simulink model "Discrete_Time_rising_ic_verif"  (Simulink 8.4)
settings: Solver=ode45  StartTime=0.0  StopTime=10.0  RelTol=1e-3
undefined symbols (not defined in the file): DiscIntNeverNeededParam, sigbuilder_block
settings Model: Creator=Romain  LastModifiedBy=hbourbou
settings DataIOCC: SignalLoggingSaveFormat=Dataset
settings OptimizationCC: ExpressionDepthLimit=128
settings DebuggingCC: SolverPrmCheckMsg=none  FcnCallInpInsideContextMsg=EnableAllAsError  FrameProcessingCompatibilityMsg=error  StateNameClashWarn=none
settings GRTTargetCC: CombineOutputUpdateFcns=on  GRTInterface=off

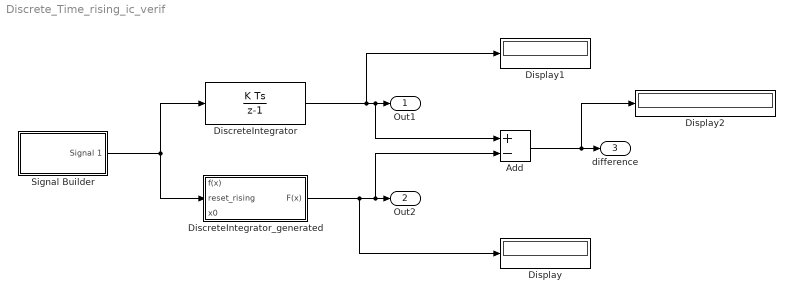
== system Discrete_Time_rising_ic_verif ==
  Add : Sum  Inputs=+-
  DiscreteIntegrator : DiscreteIntegrator  ExternalReset=rising  InitialConditionSource=external  InitialConditionSetting=State (most efficient)  SampleTime=-1  ICPrevOutput=DiscIntNeverNeededParam  ICPrevScaledInput=DiscIntNeverNeededParam
  DiscreteIntegrator_generated : Subsystem  TreatAsAtomicUnit=on
  Display : Display
  Display1 : Display
  Display2 : Display
  Signal Builder : Subsystem  Tag=STV Subsys  LoadFcn=sigbuilder_block('load');  StartFcn=sigbuilder_block('start');  StopFcn=sigbuilder_block('stop');  ClipboardFcn=sigbuilder_block('clipboard');  mask(Sigbuilder block){}
      mask help: Simulink:masks:SigbuilderBlock_MD
      mask init:
      | if ~strcmp(get_param(bdroot(gcbh),'SimulationStatus'),'stopped') tuvar = sigbuilder_block('maskInit'); end
      settings: CopyFcn=sigbuilder_block('copy');  DeleteFcn=sigbuilder_block('delete');  ModelCloseFcn=sigbuilder_block('modelClose');  PreSaveFcn=sigbuilder_block('preSave');  PauseFcn=sigbuilder_block('pause');  ContinueFcn=sigbuilder_block('continue');  NameChangeFcn=sigbuilder_block('namechange');  OpenFcn=sigbuilder_block('open',[437.6 199.2 550.4 400 ]);  CloseFcn=sigbuilder_block('close');
      mask Display: plot(0, 0, 100, 100,[2, 2, 32, 32, 2], [68, 8, 8, 68, 68],[32, 2], [38, 38], [32, 19, 2],[53, 60, 44], [32, 17, 17, 2],[16, 16, 31, 31]);txt = getActiveGroup(gcbh);text(2, 100, txt,'verticalAlignment', 'top');
  Out1 : Outport
  Out2 : Outport  Port=2
  difference : Outport  Port=3
  wires:
  Signal Builder/1(Signal 1) -> DiscreteIntegrator_generated/2(reset_rising), DiscreteIntegrator/2
  DiscreteIntegrator/1 -> Display1/1, Add/1, Out1/1
  DiscreteIntegrator_generated/1(F(x)) -> Display/1, Add/2, Out2/1
  Add/1 -> Display2/1, difference/1

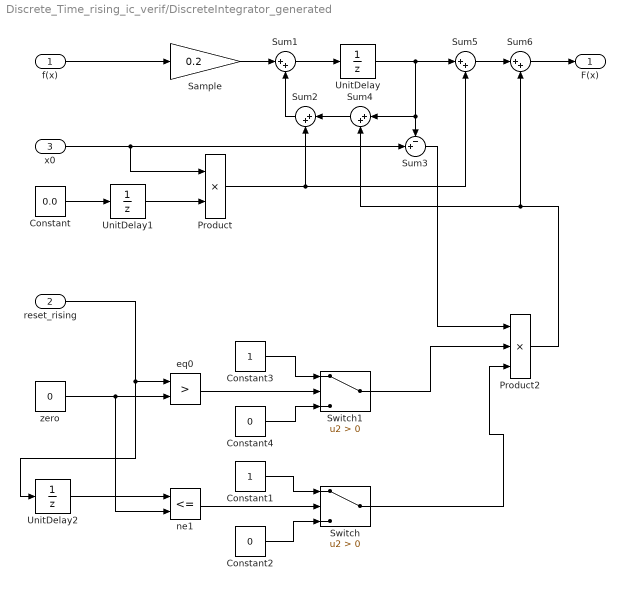
== system Discrete_Time_rising_ic_verif/DiscreteIntegrator_generated ==
  f(x) : Inport
  reset_rising : Inport  Port=2
  x0 : Inport  Port=3
  Constant : Constant  Value=0.0  SampleTime=-1
  Constant1 : Constant
  Constant2 : Constant  Value=0
  Constant3 : Constant
  Constant4 : Constant  Value=0
  Product : Product  RndMeth=Zero
  Product2 : Product  Inputs=3  RndMeth=Zero
  Sample : Gain  Gain=0.2
  Sum1 : Sum  RequirementInfo={} %GIDa_a05c8bd0_42f8_41e0_bf3c_8908fd139648  Inputs=|++
  Sum2 : Sum  RequirementInfo={} %GIDa_103a92ea_c64a_4018_b9f2_065018a0b2b4  Inputs=|++
  Sum3 : Sum  RequirementInfo={} %GIDa_f39f52c6_04c5_4a92_aada_ea48be81a6b9  Inputs=-+|
  Sum4 : Sum  RequirementInfo={} %GIDa_be87eb41_9fbd_4c5f_abda_3b11b58ffb62  Inputs=|++
  Sum5 : Sum  RequirementInfo={} %GIDa_657dc7a0_20f2_42e4_80ef_5a0fd09393d0  Inputs=|++
  Sum6 : Sum  RequirementInfo={} %GIDa_996e85b9_1925_4929_90c6_2322b6191041  Inputs=|++  SampleTime=0.2
  Switch : Switch  Criteria=u2 > Threshold
  Switch1 : Switch  Criteria=u2 > Threshold
  UnitDelay : UnitDelay  SampleTime=0.2
  UnitDelay1 : UnitDelay  InitialCondition=1  SampleTime=0.2
  UnitDelay2 : UnitDelay  SampleTime=0.2
  eq0 : RelationalOperator  Operator=>  OutDataTypeStr=boolean
  ne1 : RelationalOperator  Operator=<=  OutDataTypeStr=boolean
  zero : Constant  Value=0  SampleTime=-1
  F(x) : Outport  RequirementInfo={} %GIDa_dc32e211_828a_42c8_a49f_0942428b3921
  wires:
  Sum1/1 -> UnitDelay/1
  Sample/1 -> Sum1/1
  UnitDelay/1 -> Sum5/1, Sum3/1, Sum4/1
  Sum2/1 -> Sum1/2
  Product/1 -> Sum5/2, Sum2/2
  UnitDelay1/1 -> Product/2
  Constant/1 -> UnitDelay1/1
  x0/1 -> Product/1, Sum3/2
  reset_rising/1 -> UnitDelay2/1, eq0/1
  UnitDelay2/1 -> ne1/1
  Sum3/1 -> Product2/1
  zero/1 -> ne1/2, eq0/2
  Sum4/1 -> Sum2/1
  Product2/1 -> Sum6/2, Sum4/2
  f(x)/1 -> Sample/1
  Sum5/1 -> Sum6/1
  Sum6/1 -> F(x)/1
  ne1/1 -> Switch/2
  Constant1/1 -> Switch/1
  Constant2/1 -> Switch/3
  Switch/1 -> Product2/3
  eq0/1 -> Switch1/2
  Constant3/1 -> Switch1/1
  Constant4/1 -> Switch1/3
  Switch1/1 -> Product2/2

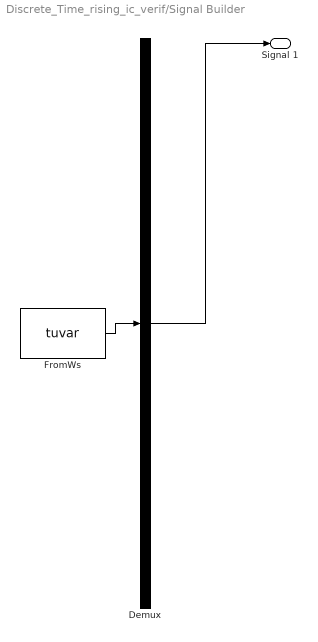
== system Discrete_Time_rising_ic_verif/Signal Builder ==
  Demux : Demux  Tag=STV Demux  Outputs=1
  FromWs : FromWorkspace  Tag=STV FromWs  VariableName=tuvar  SampleTime=0  SigBuilderData=DataTag0  VnvData=DataTag1
      SigBuilderData=|
      | common.afterFinalStr = 'Extrapolate'
      | common.sampleTime = 0
      | dataSet.timeRange = [0 10]
      | dataSet.name = 'Group 1'
      | sbobj.Groups.Name = 'Group 1'
      | sbobj.Groups.Signals.Name = 'Signal 1'
      | sbobj.Groups.Signals.XData = [0 4 4 6 6 10]
      | sbobj.Groups.Signals.YData = [0 0.99 1 0.3 0.26 0]
  Signal 1 : Outport  Tag=STV Outport
  wires:
  Demux/1 -> Signal 1/1
  FromWs/1 -> Demux/1
